simulink model "Input_Reordering"  (Simulink 7.0)
settings: Solver=FixedStepDiscrete  StartTime=0.0  StopTime=10.0  RelTol=1e-3
InitFcn:
  | %% DSPBuilder Start
  | alt_dspbuilder_update_model(bdroot)
  | %% DSPBuilder End
libraries: allblocks_alteradspbuilder2 x16
settings Model: Creator=davlin  LastModifiedBy=davlin

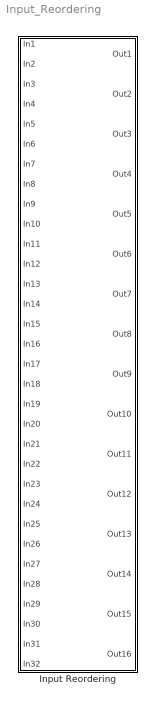
== system Input_Reordering ==
  Input Reordering : Subsystem  mask(Input Reordering - Custom Blocks){pipeline_level=0}
      mask prompts: pipeline_level "Pipeline Level:"
      mask help: This block reorders the output of the shift register.

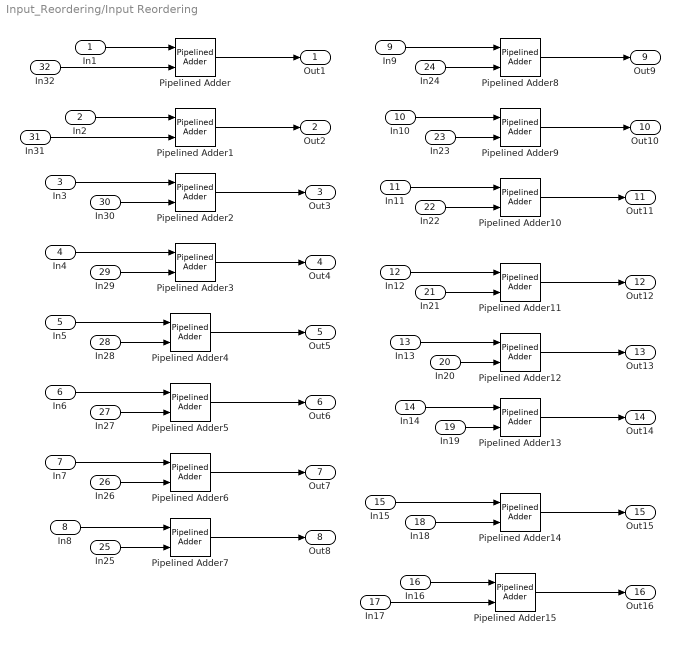
== system Input_Reordering/Input Reordering ==
  In1 : Inport  OutDataType=sfix(16)  OutScaling=2^0
  In2 : Inport  Port=2  OutDataType=sfix(16)  OutScaling=2^0
  In3 : Inport  Port=3  OutDataType=sfix(16)  OutScaling=2^0
  In4 : Inport  Port=4  OutDataType=sfix(16)  OutScaling=2^0
  In5 : Inport  Port=5  OutDataType=sfix(16)  OutScaling=2^0
  In6 : Inport  Port=6  OutDataType=sfix(16)  OutScaling=2^0
  In7 : Inport  Port=7  OutDataType=sfix(16)  OutScaling=2^0
  In8 : Inport  Port=8  OutDataType=sfix(16)  OutScaling=2^0
  In9 : Inport  Port=9  OutDataType=sfix(16)  OutScaling=2^0
  In10 : Inport  Port=10  OutDataType=sfix(16)  OutScaling=2^0
  In11 : Inport  Port=11  OutDataType=sfix(16)  OutScaling=2^0
  In12 : Inport  Port=12  OutDataType=sfix(16)  OutScaling=2^0
  In13 : Inport  Port=13  OutDataType=sfix(16)  OutScaling=2^0
  In14 : Inport  Port=14  OutDataType=sfix(16)  OutScaling=2^0
  In15 : Inport  Port=15  OutDataType=sfix(16)  OutScaling=2^0
  In16 : Inport  Port=16  OutDataType=sfix(16)  OutScaling=2^0
  In17 : Inport  Port=17  OutDataType=sfix(16)  OutScaling=2^0
  In18 : Inport  Port=18  OutDataType=sfix(16)  OutScaling=2^0
  In19 : Inport  Port=19  OutDataType=sfix(16)  OutScaling=2^0
  In20 : Inport  Port=20  OutDataType=sfix(16)  OutScaling=2^0
  In21 : Inport  Port=21  OutDataType=sfix(16)  OutScaling=2^0
  In22 : Inport  Port=22  OutDataType=sfix(16)  OutScaling=2^0
  In23 : Inport  Port=23  OutDataType=sfix(16)  OutScaling=2^0
  In24 : Inport  Port=24  OutDataType=sfix(16)  OutScaling=2^0
  In25 : Inport  Port=25  OutDataType=sfix(16)  OutScaling=2^0
  In26 : Inport  Port=26  OutDataType=sfix(16)  OutScaling=2^0
  In27 : Inport  Port=27  OutDataType=sfix(16)  OutScaling=2^0
  In28 : Inport  Port=28  OutDataType=sfix(16)  OutScaling=2^0
  In29 : Inport  Port=29  OutDataType=sfix(16)  OutScaling=2^0
  In30 : Inport  Port=30  OutDataType=sfix(16)  OutScaling=2^0
  In31 : Inport  Port=31  OutDataType=sfix(16)  OutScaling=2^0
  In32 : Inport  Port=32  OutDataType=sfix(16)  OutScaling=2^0
  Pipelined Adder{,1..15} (16 alike) : allblocks_alteradspbuilder2/Pipelined Adder  BusType=Signed Integer  bwl=12  bwr=0  pipeline=pipeline_level  pipeline_display=0  AddSubDirection=ADD  use_cin=off  use_ovl=off  use_addsub=off  use_ena=off  use_aclr=off
  Out1 : Outport  OutDataType=sfix(16)  OutScaling=2^0
  Out2 : Outport  Port=2  OutDataType=sfix(16)  OutScaling=2^0
  Out3 : Outport  Port=3  OutDataType=sfix(16)  OutScaling=2^0
  Out4 : Outport  Port=4  OutDataType=sfix(16)  OutScaling=2^0
  Out5 : Outport  Port=5  OutDataType=sfix(16)  OutScaling=2^0
  Out6 : Outport  Port=6  OutDataType=sfix(16)  OutScaling=2^0
  Out7 : Outport  Port=7  OutDataType=sfix(16)  OutScaling=2^0
  Out8 : Outport  Port=8  OutDataType=sfix(16)  OutScaling=2^0
  Out9 : Outport  Port=9  OutDataType=sfix(16)  OutScaling=2^0
  Out10 : Outport  Port=10  OutDataType=sfix(16)  OutScaling=2^0
  Out11 : Outport  Port=11  OutDataType=sfix(16)  OutScaling=2^0
  Out12 : Outport  Port=12  OutDataType=sfix(16)  OutScaling=2^0
  Out13 : Outport  Port=13  OutDataType=sfix(16)  OutScaling=2^0
  Out14 : Outport  Port=14  OutDataType=sfix(16)  OutScaling=2^0
  Out15 : Outport  Port=15  OutDataType=sfix(16)  OutScaling=2^0
  Out16 : Outport  Port=16  OutDataType=sfix(16)  OutScaling=2^0
  wires:
  In1/1 -> Pipelined Adder/1
  In32/1 -> Pipelined Adder/2
  In2/1 -> Pipelined Adder1/1
  In31/1 -> Pipelined Adder1/2
  In3/1 -> Pipelined Adder2/1
  In4/1 -> Pipelined Adder3/1
  In5/1 -> Pipelined Adder4/1
  In6/1 -> Pipelined Adder5/1
  In7/1 -> Pipelined Adder6/1
  In8/1 -> Pipelined Adder7/1
  In9/1 -> Pipelined Adder8/1
  In11/1 -> Pipelined Adder10/1
  In12/1 -> Pipelined Adder11/1
  In13/1 -> Pipelined Adder12/1
  In14/1 -> Pipelined Adder13/1
  In15/1 -> Pipelined Adder14/1
  In10/1 -> Pipelined Adder9/1
  In16/1 -> Pipelined Adder15/1
  In17/1 -> Pipelined Adder15/2
  In18/1 -> Pipelined Adder14/2
  In19/1 -> Pipelined Adder13/2
  In20/1 -> Pipelined Adder12/2
  In21/1 -> Pipelined Adder11/2
  In22/1 -> Pipelined Adder10/2
  In23/1 -> Pipelined Adder9/2
  In24/1 -> Pipelined Adder8/2
  In25/1 -> Pipelined Adder7/2
  In26/1 -> Pipelined Adder6/2
  In27/1 -> Pipelined Adder5/2
  In28/1 -> Pipelined Adder4/2
  In29/1 -> Pipelined Adder3/2
  In30/1 -> Pipelined Adder2/2
  Pipelined Adder/1 -> Out1/1
  Pipelined Adder1/1 -> Out2/1
  Pipelined Adder2/1 -> Out3/1
  Pipelined Adder3/1 -> Out4/1
  Pipelined Adder4/1 -> Out5/1
  Pipelined Adder5/1 -> Out6/1
  Pipelined Adder6/1 -> Out7/1
  Pipelined Adder7/1 -> Out8/1
  Pipelined Adder8/1 -> Out9/1
  Pipelined Adder9/1 -> Out10/1
  Pipelined Adder10/1 -> Out11/1
  Pipelined Adder15/1 -> Out16/1
  Pipelined Adder14/1 -> Out15/1
  Pipelined Adder13/1 -> Out14/1
  Pipelined Adder12/1 -> Out13/1
  Pipelined Adder11/1 -> Out12/1
